simulink model "c_station_v3"  (R2019a)
settings: Solver=VariableStepAuto  StartTime=0.0  StopTime=604800  MaxStep=3600  RelTol=1e-3  AbsTol=1e-3  EnableMultiTasking=on
StopFcn:
  | displayGasParameters(gasPressures);
values from neighbouring files (symbols this model uses):
  conf = gasConfig()    [gas_v1.m]
  valveControlFlag = "on"    [gas_v1.m]
undefined symbols (not defined in the file or in its folder): lineParm, loadParm, valveParm
libraries: gasLibrary x25, fl_lib x19, nesl_utility x11, SimscapeFluids_lib x1
(part 1 of 3)
settings Model: Creator=dzimm  LastModifiedBy=brandt
settings SolverCC: AutoScaleAbsTol=off
settings DataIOCC: LimitDataPoints=on  MaxDataPoints=10000  ReturnWorkspaceOutputs=off
settings OptimizationCC: LifeSpan=inf
settings DebuggingCC: AllowSymbolicDim=off  PregeneratedLibrarySubsystemCodeDiagnostic=none  SFUnexpectedBacktrackingDiag=warning  SFNoUnconditionalDefaultTransitionDiag=warning  SFExecutionAtInitializationDiag=none  ArithmeticOperatorsInVariantConditions=warning
settings SFSimCC: SimUseLocalCustomCode=off
settings RTWCC: RTWUseLocalCustomCode=off
settings CodeAppCC: StateflowObjectComments=on
settings GRTTargetCC: TargetLangStandard=C89/C90 (ANSI)  GeneratePreprocessorConditionals=Disable all
settings ConfigComp: CovMetricSettings=dw  CovHtmlReporting=on  CovSaveCumulativeToWorkspaceVar=on  CovSaveSingleToWorkspaceVar=on  CovExternalEMLEnable=off  CovSFcnEnable=off
settings SimscapeCC: SimscapeLogType=all  SimscapeLogOpenViewer=on  SimscapeLogLimitData=off  SimscapeLogDataHistory=10000  SimscapeUseOperatingPoints=on  SimscapeOperatingPoint=op

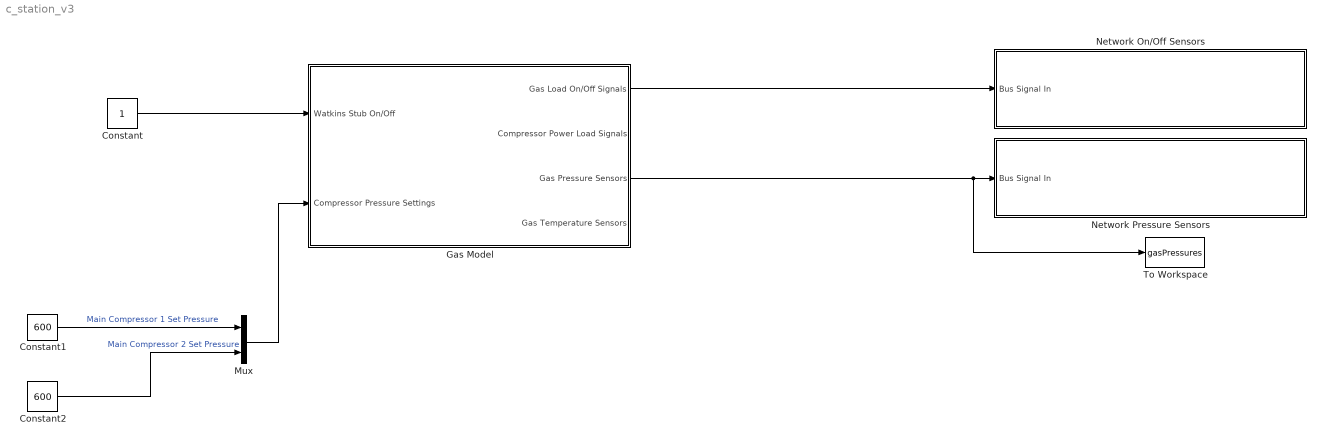
== system c_station_v3 ==
  Constant : Constant
  Constant1 : Constant  Value=600
  Constant2 : Constant  Value=600
  Gas Model : Subsystem
  Mux : Mux  Inputs=2
  Network On/Off Sensors : Subsystem
  Network Pressure Sensors : Subsystem
  To Workspace : ToWorkspace  VariableName=gasPressures  SaveFormat=Timeseries  SampleTime=-1
  wires:
  Constant/1 -> Gas Model/1(Watkins Stub On/Off)
  Constant1/1 -> Mux/1  "Main Compressor 1 Set Pressure"
  Constant2/1 -> Mux/2  "Main Compressor 2 Set Pressure"
  Mux/1 -> Gas Model/2(Compressor Pressure Settings)
  Gas Model/3(Gas Pressure Sensors) -> Network Pressure Sensors/1(Bus Signal In), To Workspace/1
  Gas Model/1(Gas Load On/Off Signals) -> Network On/Off Sensors/1(Bus Signal In)
